simulink model "DVLineairelinmod"  (Simulink 8.5)
settings: Solver=ode45  StartTime=0.0  StopTime=6  RelTol=1e-3
values from neighbouring files (symbols this model uses):
  ba = 11.9097222222    [Correcteur.mat]    (also in DVinitialisation.m; QFT.m = ro*Sx*Cx*Vxe)
  br = 0.001    [Correcteur.mat]    (also in DVinitialisation.m; QFT.m)
  brr = 0.003052    [Correcteur.mat]    (also in DVinitialisation.m; QFT.m = 2*lambda2*m*g*Vxe)
  Cm0 = 42.8155296593    [Correcteur.mat]    (also in DVinitialisation.m = r0*FXE+br*W0; QFT.m = r0*FXE+br*W0)
  cxe = 56680.57116    [Correcteur.mat]    (also in DVinitialisation.m = cx*100; QFT.m = 100*mu*(b3*Z^2+b4*Z)*exp(-b5*Z))
  J = 1    [Correcteur.mat]    (also in DVinitialisation.m; QFT.m)
  K = 125    [Correcteur.mat]    (also in DVinitialisation.m; PIDF_Design.m = K/M; QFT.m)
  m = 200    [Correcteur.mat]    (also in DVinitialisation.m; QFT.m = var1(i1))
  mufre = -0.0515581949912    [Correcteur.mat]    (also in DVinitialisation.m = -(r0*W0e)/(Vxe*Vxe); QFT.m = -(r0*W0)/(Vxe*Vxe))
  nfre = 0.0154285714286    [Correcteur.mat]    (also in DVinitialisation.m; QFT.m = r0/Vxe)
  r0 = 0.3    [Correcteur.mat]    (also in DVinitialisation.m; QFT.m)
  Vx0 = 19.4444444444    [Correcteur.mat]    (also in DVinitialisation.m; QFT.m = var3(i3))
  W0 = 64.9781778438    [Correcteur.mat]    (also in DVinitialisation.m = 1/r0*(Vx0/(1-(Te/100))); QFT.m = 1/r0*(Vx0/(1-(Te/100))))
settings Model: Creator=StephaneBarroso  LastModifiedBy=StephaneBarroso
settings DataIOCC: SignalLoggingSaveFormat=Dataset
settings OptimizationCC: ExpressionDepthLimit=128
settings DebuggingCC: UnderspecifiedInitializationDetection=Simplified  MergeDetectMultiDrivingBlocksExec=error  FcnCallInpInsideContextMsg=EnableAllAsError  StateNameClashWarn=none
settings GRTTargetCC: CombineOutputUpdateFcns=on  GRTInterface=off

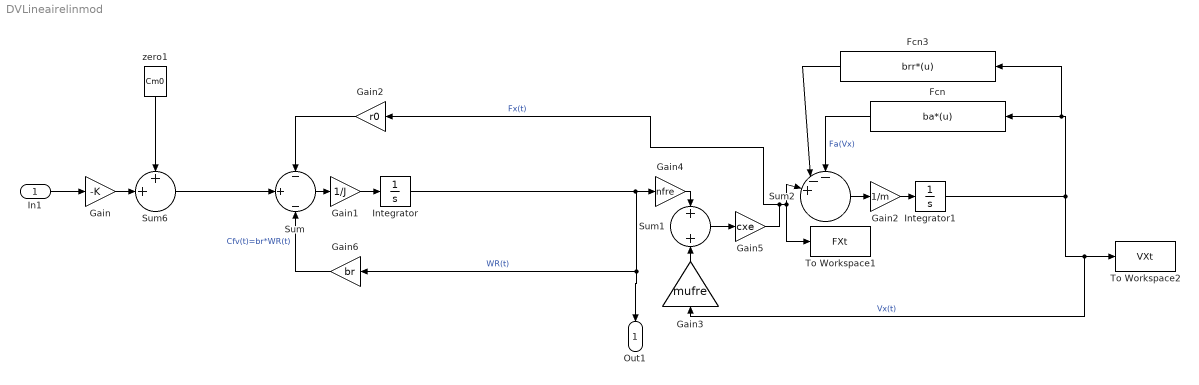
== system DVLineairelinmod ==
  In1 : Inport
  Fcn : Fcn  Expr=ba*(u)
  Fcn3 : Fcn  Expr=brr*(u)
  Gain : Gain  Gain=-K
  Gain1 : Gain  Gain=1/J
  Gain2 : Gain  Gain=r0
  "Gain2 " : Gain  Gain=1/m
  Gain3 : Gain  Gain=mufre
  Gain4 : Gain  Gain=nfre
  Gain5 : Gain  Gain=cxe
  Gain6 : Gain  Gain=br
  Integrator : Integrator  InitialCondition=W0
  Integrator1 : Integrator  InitialCondition=Vx0
  Sum : Sum  Inputs=-|+|-
  Sum1 : Sum
  Sum2 : Sum  Inputs=--+|||
  Sum6 : Sum  Inputs=++|
  To Workspace1 : ToWorkspace  VariableName=FXt  SaveFormat=Timeseries  SampleTime=-1
  To Workspace2 : ToWorkspace  VariableName=VXt  SaveFormat=Timeseries  SampleTime=-1
  zero1 : Constant  Value=Cm0
  Out1 : Outport
  wires:
  zero1/1 -> Sum6/1
  Gain/1 -> Sum6/2
  In1/1 -> Gain/1
  Gain4/1 -> Sum1/1
  Gain3/1 -> Sum1/2
  Sum1/1 -> Gain5/1
  Gain2/1 -> Sum/1
  Integrator/1 -> Gain4/1, Gain6/1, Out1/1  "WR(t)"
  Gain1/1 -> Integrator/1
  Integrator1/1 -> To Workspace2/1, Gain3/1, Fcn3/1, Fcn/1  "Vx(t)"
  "Gain2 "/1 -> Integrator1/1
  Gain6/1 -> Sum/3  "Cfv(t)=br*WR(t)"
  Fcn3/1 -> Sum2/2
  Sum2/1 -> "Gain2 "/1
  Fcn/1 -> Sum2/1  "Fa(Vx)"
  Sum/1 -> Gain1/1
  Sum6/1 -> Sum/2
  Gain5/1 -> Gain2/1, Sum2/3, To Workspace1/1  "Fx(t)"
